simulink model "Stockton_Project1_model2"  (R2014a)
settings: Solver=ode3  StartTime=0.0  StopTime=10  FixedStep=0.01  RelTol=1e-7
values from neighbouring files (symbols this model uses):
  den = conv(CE_lp,CE_sp)    [Final.m]    (also in Fuzzy_PID_Comp.m = dens{i}; Stockton_Project1.m = [230.6,2508,2161,1406,63.04,32.01])
  num = -4.516*conv([1 -0.008],[1 0.506])    [Final.m]    (also in Fuzzy_PID_Comp.m = nums{i}; Stockton_Project1.m = [3361,1357,102.2])
libraries: fuzblock x1
settings Model: Creator=nick  LastModifiedBy=nick
settings SolverCC: ZeroCrossControl=DisableAll  ZeroCrossAlgorithm=Adaptive
settings DebuggingCC: SolverPrmCheckMsg=none

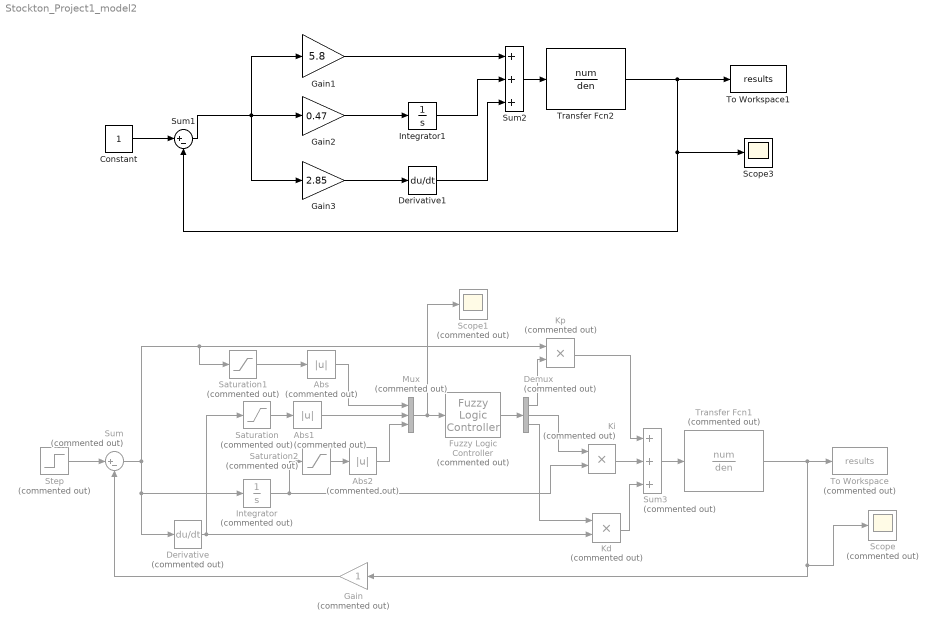
== system Stockton_Project1_model2 ==
  Abs : Abs  Commented=on
  Abs1 : Abs  Commented=on
  Abs2 : Abs  Commented=on
  Constant : Constant
  Demux : Demux  Commented=on  Outputs=3
  Derivative : Derivative  Commented=on
  Derivative1 : Derivative
  Fuzzy Logic Controller : fuzblock/Fuzzy Logic  Controller  Commented=on  fis=fis
  Gain : Gain  Commented=on
  Gain1 : Gain  Gain=5.8
  Gain2 : Gain  Gain=0.47
  Gain3 : Gain  Gain=2.85
  Integrator : Integrator  Commented=on
  Integrator1 : Integrator
  Kd : Product  Commented=on
  Ki : Product  Commented=on
  Kp : Product  Commented=on
  Mux : Mux  Commented=on  Inputs=3
  Saturation : Saturate  Commented=on  UpperLimit=19.9  LowerLimit=-19.9
  Saturation1 : Saturate  Commented=on  UpperLimit=19.9  LowerLimit=-19.9
  Saturation2 : Saturate  Commented=on  UpperLimit=19.9  LowerLimit=-19.9
  Scope : Scope  Commented=on
      settings: YMin=-2.25e+50  YMax=0
  Scope1 : Scope  Commented=on
      settings: YMin=0  YMax=20
  Scope3 : Scope
      settings: SaveName=ScopeData3
  Step : Step  Commented=on  Time=0  SampleTime=0
  Sum : Sum  Commented=on  Inputs=|+-
  Sum1 : Sum  Inputs=|+-
  Sum2 : Sum  Inputs=+++
  Sum3 : Sum  Commented=on  Inputs=+++
  To Workspace : ToWorkspace  Commented=on  VariableName=results  SaveFormat=Timeseries  SampleTime=-1
  To Workspace1 : ToWorkspace  VariableName=results  SaveFormat=Timeseries  SampleTime=-1
  Transfer Fcn1 : TransferFcn  Commented=on  Numerator=num  Denominator=den
  Transfer Fcn2 : TransferFcn  Numerator=num  Denominator=den
  wires:
  Gain/1 -> Sum/2
  Step/1 -> Sum/1
  Constant/1 -> Sum1/1
  Transfer Fcn2/1 -> To Workspace1/1, Scope3/1, Sum1/2
  Kp/1 -> Sum3/1
  Gain1/1 -> Sum2/1
  Mux/1 -> Scope1/1, Fuzzy Logic Controller/1
  Fuzzy Logic Controller/1 -> Demux/1
  Abs1/1 -> Mux/2
  Abs/1 -> Mux/1
  Kd/1 -> Sum3/3
  Ki/1 -> Sum3/2
  Sum/1 -> Derivative/1, Integrator/1, Kp/1, Saturation1/1
  Demux/1 -> Kp/2
  Demux/2 -> Ki/1
  Demux/3 -> Kd/1
  Integrator/1 -> Ki/2, Saturation2/1
  Derivative/1 -> Kd/2, Saturation/1
  Integrator1/1 -> Sum2/2
  Gain2/1 -> Integrator1/1
  Derivative1/1 -> Sum2/3
  Sum1/1 -> Gain3/1, Gain2/1, Gain1/1
  Gain3/1 -> Derivative1/1
  Sum2/1 -> Transfer Fcn2/1
  Transfer Fcn1/1 -> Gain/1, Scope/1, To Workspace/1
  Sum3/1 -> Transfer Fcn1/1
  Saturation/1 -> Abs1/1
  Saturation1/1 -> Abs/1
  Abs2/1 -> Mux/3
  Saturation2/1 -> Abs2/1
